simulink model "linearized_STeVe"  (R2024b)
settings: Solver=ode8  StartTime=0.0  StopTime=30  FixedStep=0.0001  RelTol=1e-3
libraries: simulink_extras x6, aerolibactuator x2
settings Model: Creator=jonno  LastModifiedBy=jonno

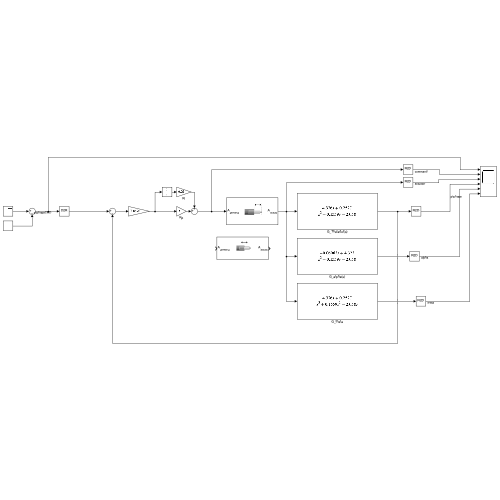
[thumbnail: Simulink's stored preview of the top-level diagram]
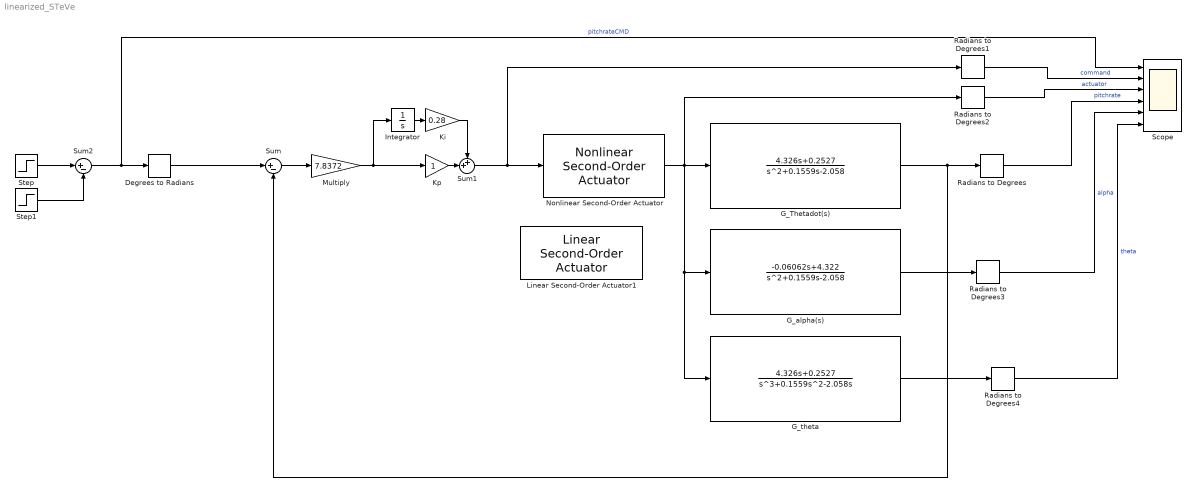
== system linearized_STeVe ==
  Degrees to Radians : simulink_extras/Transformations/Degrees to Radians
  G_Thetadot(s) : TransferFcn  Numerator=[4.326 0.2527]  Denominator=[1 0.1559 -2.058]
  G_alpha(s) : TransferFcn  Numerator=[-0.06062 4.322]  Denominator=[1 0.1559 -2.058]
  G_theta : TransferFcn  Numerator=[4.326 0.2527]  Denominator=[1 0.1559 -2.058 0]
  Integrator : Integrator
  Ki : Gain  Gain=0.28
  Kp : Gain
  Linear Second-Order Actuator1 : aerolibactuator/Linear Second-Order Actuator  wn_fin=62  z_fin=0.5858  fin_act_0=0  fin_act_vel=0
  Multiply : Gain  Gain=7.8372
  Nonlinear Second-Order Actuator : aerolibactuator/Nonlinear Second-Order Actuator  wn_fin=62  z_fin=0.585  fin_max=6*pi/180  fin_min=-6*pi/180  fin_maxrate=50*pi/180  fin_act_0=0  fin_act_vel=0
  Radians to Degrees{,1..4} (5 alike) : simulink_extras/Transformations/Radians to Degrees
  Scope : Scope  NumInputPorts=6
  Step : Step  After=5  SampleTime=0
  Step1 : Step  Time=2  After=5  SampleTime=0
  Sum : Sum  Inputs=|+-
  Sum1 : Sum  Inputs=++|
  Sum2 : Sum  Inputs=|+-
  wires:
  Sum2/1 -> Scope/1, Degrees to Radians/1  "pitchrateCMD"
  Degrees to Radians/1 -> Sum/1
  Sum/1 -> Multiply/1
  Integrator/1 -> Ki/1
  Kp/1 -> Sum1/2
  Ki/1 -> Sum1/1
  Sum1/1 -> Nonlinear Second-Order Actuator/1, Radians to Degrees1/1
  Radians to Degrees/1 -> Scope/4  "pitchrate"
  Multiply/1 -> Integrator/1, Kp/1
  G_Thetadot(s)/1 -> Radians to Degrees/1, Sum/2
  Nonlinear Second-Order Actuator/1 -> G_theta/1, G_alpha(s)/1, Radians to Degrees2/1, G_Thetadot(s)/1
  Radians to Degrees1/1 -> Scope/2  "command"
  Radians to Degrees2/1 -> Scope/3  "actuator"
  G_alpha(s)/1 -> Radians to Degrees3/1
  Radians to Degrees3/1 -> Scope/5  "alpha"
  Step/1 -> Sum2/1
  G_theta/1 -> Radians to Degrees4/1
  Radians to Degrees4/1 -> Scope/6  "theta"
  Step1/1 -> Sum2/2
